simulink subsystem "s_function_quantile_effort_controller"  (R2024b)
settings: Solver=VariableStepAuto  StartTime=0.0  StopTime=10.0  RelTol=1e-3
undefined symbols (not defined in the file): const_brake, controller_rate
settings Model: Creator=yevge  LastModifiedBy=agaydos

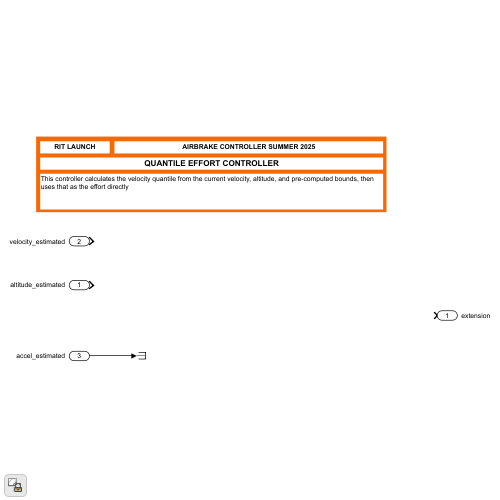
[thumbnail: Simulink's stored preview of the top-level diagram]
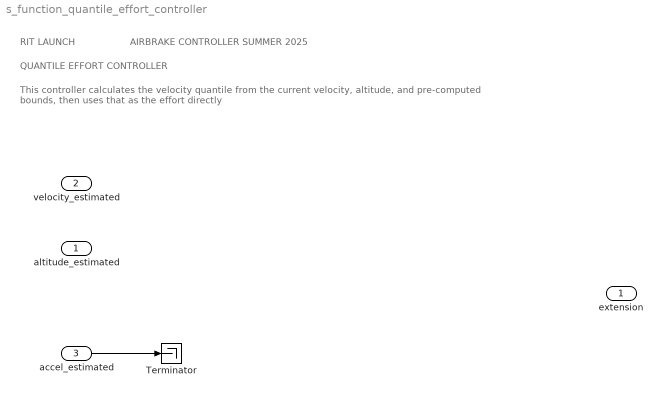
== system s_function_quantile_effort_controller ==
  note: QUANTILE EFFORT CONTROLLER
  note: This controller calculates the velocity quantile from the current velocity, altitude, and pre-computed bounds, then uses that as the effort directly
  note: RIT LAUNCH
  note: AIRBRAKE CONTROLLER SUMMER 2025
  altitude_estimated : Inport  Unit=m  PortDimensions=1
  velocity_estimated : Inport  Port=2  Unit=m/s  PortDimensions=1
  accel_estimated : Inport  Port=3  Unit=m/s^2  PortDimensions=1
  Terminator : Terminator
  extension : Outport  Unit=1  PortDimensions=1  SampleTime=1/controller_rate  InitialOutput=const_brake
  wires:
  accel_estimated/1 -> Terminator/1
